simulink model "hdv_ctrl"  (R2026a)
settings: Solver=ode23tb  StopTime=simulation_length  MaxStep=tsample
undefined symbols (not defined in the file): available_torque, eta_v_m, eta_v_p, omega_e_rpm_ref, omega_l_max_rpm, R_tg, rpm, tau_load, tau_load_max, tsample, v_track1_ref, v_track2_ref
libraries: nesl_utility x20, fl_lib x13, linear_swashplate_ctrl_lib x4, variable_displacement_motor_lib x2, variable_displacement_pump_lib x2, flexshaft_lib x2, gear_lib x2, sl_discontinuities x2, engine_speed_ctrl_lib x1, engine_lib x1
settings Model: SimulationMode=accelerator  Creator=dbagn  LastModifiedBy=dbagn
settings SimscapeCC: SimscapeNominalValues="[{\"value\":\"1\",\"unit\":\"A\"},{\"value\":\"1\",\"unit\":\"bar\"},{\"value\":\"1\",\"unit\":\"cm^2\"},{\"value\":\"1\",\"unit\":\"cm^3/s\"},{\"value\":\"1\",\"unit\":\"kJ/kg\"},{\"value\":\"1\",\"unit\":\"kW\"},{\"value\":\"1\",\"unit\":\"l\"},{\"value\":\"1\",\"unit\":\"N\"},{\"value\":\"1\",\"unit\":\"N*m\"},{\"value\":\"1\",\"unit\":\"V\"}]"  SimscapeLogType=none  SimscapeLogDataHistory=5000.0

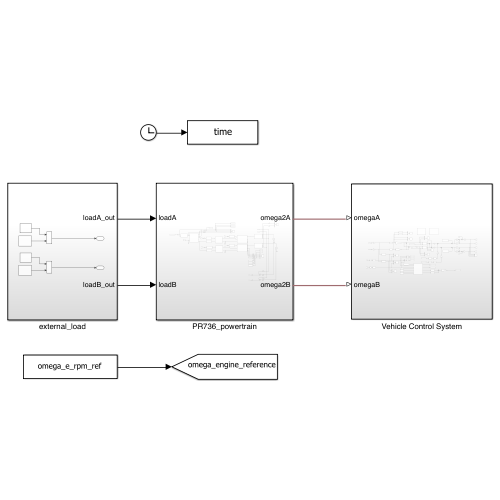
[thumbnail: Simulink's stored preview of the top-level diagram]
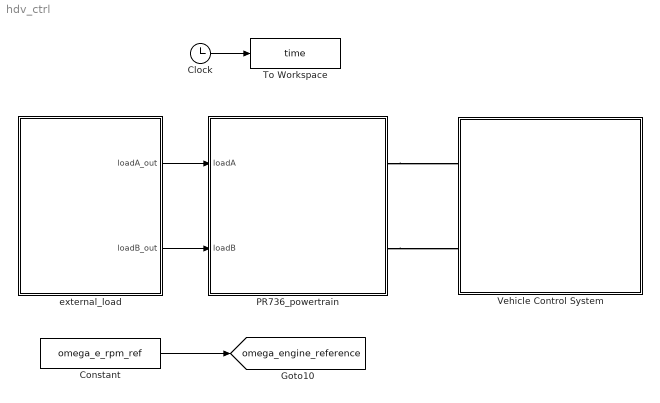
== system hdv_ctrl ==
  Clock : Clock
  Constant : Constant  Value=omega_e_rpm_ref
  PR736_powertrain : Subsystem
  To Workspace : ToWorkspace  VariableName=time  SampleTime=tsample
      settings: MaxDataPoints=Nsample
  Vehicle Control System : Subsystem
  external_load : Subsystem
  tag scope: omega_engine_reference=global
  wires:
  Clock/1 -> To Workspace/1
  Constant/1 -> [omega_engine_reference]
  external_load/2(loadB_out) -> PR736_powertrain/2(loadB)
  external_load/1(loadA_out) -> PR736_powertrain/1(loadA)
  connections:
  PR736_powertrain/RConn1 -- Vehicle Control System/LConn1
  PR736_powertrain/RConn2 -- Vehicle Control System/LConn2

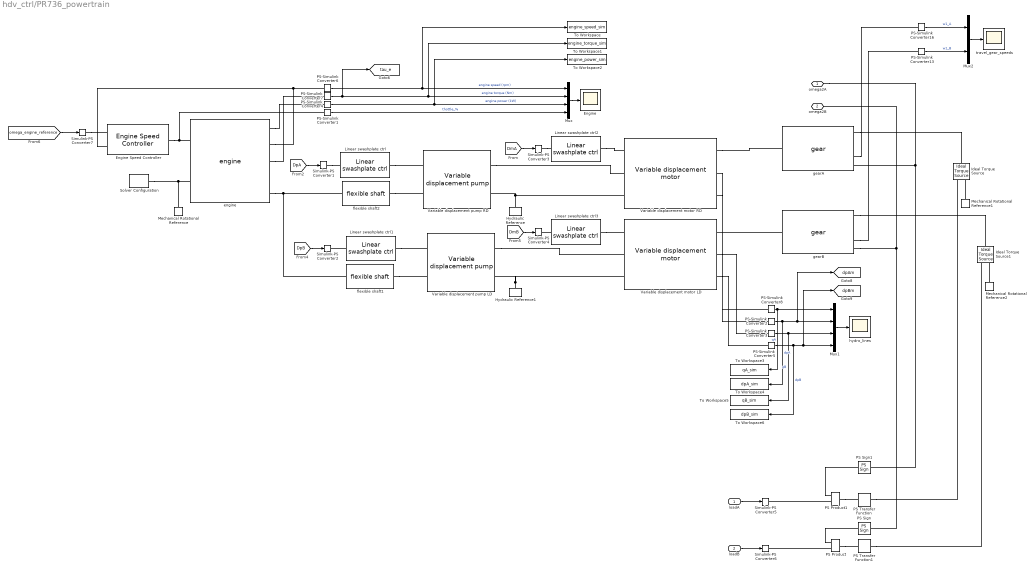
== system hdv_ctrl/PR736_powertrain ==
  loadA : Inport
  loadB : Inport  Port=2
  Engine : Scope
      settings: SampleTime=tsample  ActiveDisplayYMinimum=-336.80549  ActiveDisplayYMaximum=2213.60139
  Engine Speed Controller : engine_speed_ctrl_lib/Engine Speed Controller  kp=0.25 s  kint=2  kd=0 s^2  t_out_specify=off  t_out_priority=None  t_out=0  t_out_nominal_specify=off  t_out_nominal_unit=1  t_out_nominal_value=1
  Hydraulic Reference : fl_lib/Hydraulic/Hydraulic Elements/Hydraulic Reference
  Hydraulic Reference1 : fl_lib/Hydraulic/Hydraulic Elements/Hydraulic Reference
  Ideal Torque Source : fl_lib/Mechanical/Mechanical Sources/Ideal Torque Source
  Ideal Torque Source1 : fl_lib/Mechanical/Mechanical Sources/Ideal Torque Source
  Linear swashplate ctrl : linear_swashplate_ctrl_lib/Linear swashplate ctrl  a12=1 1/s  b2=1 1/m/s  k1=100 m  k2=20.5 m  N=10 m  kv=10  xv_specify=off  xv_priority=None  xv=0 m  xv_nominal_specify=off  xv_nominal_unit=m  xv_nominal_value=1  D1_specify=off  D1_priority=None  D1=0  D1_nominal_specify=off  D1_nominal_unit=1  D1_nominal_value=1  D2_specify=off  D2_priority=None  D2=0  D2_nominal_specify=off  D2_nominal_unit=1  D2_nominal_value=1
  Linear swashplate ctrl1 : linear_swashplate_ctrl_lib/Linear swashplate ctrl  a12=1 1/s  b2=1 1/m/s  k1=100 m  k2=20.5 m  N=10 m  kv=10  xv_specify=off  xv_priority=None  xv=0 m  xv_nominal_specify=off  xv_nominal_unit=m  xv_nominal_value=1  D1_specify=off  D1_priority=None  D1=0  D1_nominal_specify=off  D1_nominal_unit=1  D1_nominal_value=1  D2_specify=off  D2_priority=None  D2=0  D2_nominal_specify=off  D2_nominal_unit=1  D2_nominal_value=1
  Linear swashplate ctrl2 : linear_swashplate_ctrl_lib/Linear swashplate ctrl  a12=1 1/s  b2=1 1/m/s  k1=100 m  k2=20.5 m  N=5 m  kv=20  xv_specify=off  xv_priority=None  xv=0 m  xv_nominal_specify=off  xv_nominal_unit=m  xv_nominal_value=1  D1_specify=off  D1_priority=None  D1=0  D1_nominal_specify=off  D1_nominal_unit=1  D1_nominal_value=1  D2_specify=off  D2_priority=None  D2=0  D2_nominal_specify=off  D2_nominal_unit=1  D2_nominal_value=1
  Linear swashplate ctrl3 : linear_swashplate_ctrl_lib/Linear swashplate ctrl  a12=1 1/s  b2=1 1/m/s  k1=100 m  k2=20.5 m  N=5 m  kv=20  xv_specify=off  xv_priority=None  xv=0 m  xv_nominal_specify=off  xv_nominal_unit=m  xv_nominal_value=1  D1_specify=off  D1_priority=None  D1=0  D1_nominal_specify=off  D1_nominal_unit=1  D1_nominal_value=1  D2_specify=off  D2_priority=None  D2=0  D2_nominal_specify=off  D2_nominal_unit=1  D2_nominal_value=1
  Mechanical Rotational Reference : fl_lib/Mechanical/Rotational Elements/Mechanical Rotational Reference
  Mechanical Rotational Reference1 : fl_lib/Mechanical/Rotational Elements/Mechanical Rotational Reference
  Mechanical Rotational Reference2 : fl_lib/Mechanical/Rotational Elements/Mechanical Rotational Reference
  Mux : Mux
  Mux1 : Mux
  Mux2 : Mux  Inputs=2
  PS Product : fl_lib/Physical Signals/Functions/PS Product
  PS Product1 : fl_lib/Physical Signals/Functions/PS Product
  PS Sign : fl_lib/Physical Signals/Nonlinear Operators/PS Sign
  PS Sign1 : fl_lib/Physical Signals/Nonlinear Operators/PS Sign
  PS Transfer Function : fl_lib/Physical Signals/Linear Operators/PS Transfer Function  transfer_function_type=foundation.enum.transfer_function_type.lag  T=1 s  T1=2 s  T2=1 s  reset_method=foundation.enum.IntegratorResetSpec.None  initial_condition_spec=foundation.enum.IntegratorICSpec.Internal  y0=0 N*m
  PS Transfer Function1 : fl_lib/Physical Signals/Linear Operators/PS Transfer Function  transfer_function_type=foundation.enum.transfer_function_type.lag  T=1 s  T1=2 s  T2=1 s  reset_method=foundation.enum.IntegratorResetSpec.None  initial_condition_spec=foundation.enum.IntegratorICSpec.Internal  y0=0 N*m
  PS-Simulink Converter1 : nesl_utility/PS-Simulink Converter  PhysicalDomain=network_engine_domain  SubClassName=ps_output  LeftPortType=input  RightPortType=output  PseudoPeriodic=off  Frequencies=[]  VectorFormat=1-D array  Unit=inherit  AffineConversion=off
  PS-Simulink Converter13 : nesl_utility/PS-Simulink Converter  PhysicalDomain=network_engine_domain  SubClassName=ps_output  LeftPortType=input  RightPortType=output  PseudoPeriodic=off  Frequencies=[]  VectorFormat=1-D array  Unit=rpm  AffineConversion=on
  PS-Simulink Converter16 : nesl_utility/PS-Simulink Converter  PhysicalDomain=network_engine_domain  SubClassName=ps_output  LeftPortType=input  RightPortType=output  PseudoPeriodic=off  Frequencies=[]  VectorFormat=1-D array  Unit=rpm  AffineConversion=on
  PS-Simulink Converter2 : nesl_utility/PS-Simulink Converter  PhysicalDomain=network_engine_domain  SubClassName=ps_output  LeftPortType=input  RightPortType=output  PseudoPeriodic=off  Frequencies=[]  VectorFormat=1-D array  Unit=bar  AffineConversion=off
  PS-Simulink Converter3 : nesl_utility/PS-Simulink Converter  PhysicalDomain=network_engine_domain  SubClassName=ps_output  LeftPortType=input  RightPortType=output  PseudoPeriodic=off  Frequencies=[]  VectorFormat=1-D array  Unit=l/min  AffineConversion=off
  PS-Simulink Converter4 : nesl_utility/PS-Simulink Converter  PhysicalDomain=network_engine_domain  SubClassName=ps_output  LeftPortType=input  RightPortType=output  PseudoPeriodic=off  Frequencies=[]  VectorFormat=1-D array  Unit=kW  AffineConversion=off
  PS-Simulink Converter5 : nesl_utility/PS-Simulink Converter  PhysicalDomain=network_engine_domain  SubClassName=ps_output  LeftPortType=input  RightPortType=output  PseudoPeriodic=off  Frequencies=[]  VectorFormat=1-D array  Unit=bar  AffineConversion=off
  PS-Simulink Converter6 : nesl_utility/PS-Simulink Converter  PhysicalDomain=network_engine_domain  SubClassName=ps_output  LeftPortType=input  RightPortType=output  PseudoPeriodic=off  Frequencies=[]  VectorFormat=1-D array  Unit=rpm  AffineConversion=off
  PS-Simulink Converter7 : nesl_utility/PS-Simulink Converter  PhysicalDomain=network_engine_domain  SubClassName=ps_output  LeftPortType=input  RightPortType=output  PseudoPeriodic=off  Frequencies=[]  VectorFormat=1-D array  Unit=inherit  AffineConversion=off
  PS-Simulink Converter8 : nesl_utility/PS-Simulink Converter  PhysicalDomain=network_engine_domain  SubClassName=ps_output  LeftPortType=input  RightPortType=output  PseudoPeriodic=off  Frequencies=[]  VectorFormat=1-D array  Unit=l/min  AffineConversion=off
  Simulink-PS Converter{1..4} (4 alike) : nesl_utility/Simulink-PS Converter  PhysicalDomain=network_engine_domain  SubClassName=ps_input  LeftPortType=input  RightPortType=output  PseudoPeriodic=off  Frequencies=[]  NoiseDistribution=none  NoiseParameters=[]  Unit=1  AffineConversion=off  FilteringAndDerivatives=provide  SimscapeFilterOrder=1  InputFilterTimeConstant=0.001  UdotUserProvided=0
  Simulink-PS Converter5 : nesl_utility/Simulink-PS Converter  PhysicalDomain=network_engine_domain  SubClassName=ps_input  LeftPortType=input  RightPortType=output  PseudoPeriodic=off  Frequencies=[]  NoiseDistribution=none  NoiseParameters=[]  Unit=N*m  AffineConversion=off  FilteringAndDerivatives=provide  SimscapeFilterOrder=1  InputFilterTimeConstant=0.001  UdotUserProvided=0
  Simulink-PS Converter6 : nesl_utility/Simulink-PS Converter  PhysicalDomain=network_engine_domain  SubClassName=ps_input  LeftPortType=input  RightPortType=output  PseudoPeriodic=off  Frequencies=[]  NoiseDistribution=none  NoiseParameters=[]  Unit=N*m  AffineConversion=off  FilteringAndDerivatives=provide  SimscapeFilterOrder=1  InputFilterTimeConstant=0.001  UdotUserProvided=0
  Simulink-PS Converter7 : nesl_utility/Simulink-PS Converter  PhysicalDomain=network_engine_domain  SubClassName=ps_input  LeftPortType=input  RightPortType=output  PseudoPeriodic=off  Frequencies=[]  NoiseDistribution=none  NoiseParameters=[]  Unit=rpm  AffineConversion=off  FilteringAndDerivatives=provide  SimscapeFilterOrder=1  InputFilterTimeConstant=0.001  UdotUserProvided=0
  Solver Configuration : nesl_utility/Solver Configuration  PhysicalDomain=network_engine_domain  SubClassName=solver  LeftPortType=input  RightPortType=generic  Tones=[]  Harmonics=[]  SimulateNoise=off  Profile=off  UseLocalSampling=off  EnableSwitchedLinearOptims=on  FrequencyDomain=off  UseCCode=off  RelTol=0.001  AbsTol=1e-06  MinStep=1e-09  ToWorkspace=off  RevertToSquareIcSolve=off  NumHomotopyIterations=100  PhasorMode=off  PhasorModeNumHarmonics=1  ConsistencySolver=NEWTON_FTOL  CanonicalOrdering=UNORDERED  OptimizeIntermediates=UNOPTIMIZED  IndexReductionMethod=DerivativeReplacement  DoDC=off  ResidualTolerance=1e-09  ConsistencyTolSource=GLOBAL  ConsistencyAbsTol=0.001  ConsistencyRelTol=0.001  ConsistencyTolFactor=0.001  UseLocalSolver=on  LocalSolverChoice=NE_BACKWARD_EULER_ADVANCER  ResolveIndetEquations=on  FunctionEvalNumThread=1  LocalSolverSampleTime=tsample  DoFixedCost=on  MaxNonlinIter=3  MaxModeIter=2  ComputeImpulses=off  ImpulseIterations=2  LinearAlgebra=auto  LinearAlgebraNumThread=0  EquationFormulation=NE_TIME_EF  DelaysMemoryBudget=1024  AutomaticFiltering=on  FilteringTimeConstant=tsample  PartitionStorageMethod=AS_NEEDED  PartitionMemoryBudget=1024  PartitionMethod=ROBUST  MultibodyUseLocalSolver=off  MultibodyLocalSolverChoice=ODE1  MultibodyLocalSolverSampleTime=0.001
  To Workspace : ToWorkspace  VariableName=engine_speed_sim  SampleTime=tsample
      settings: MaxDataPoints=Nsample
  To Workspace1 : ToWorkspace  VariableName=engine_torque_sim  SampleTime=tsample
      settings: MaxDataPoints=Nsample
  To Workspace2 : ToWorkspace  VariableName=engine_power_sim  SampleTime=tsample
      settings: MaxDataPoints=Nsample
  To Workspace3 : ToWorkspace  VariableName=qA_sim  SampleTime=tsample
      settings: MaxDataPoints=Nsample
  To Workspace4 : ToWorkspace  VariableName=dpA_sim  SampleTime=tsample
      settings: MaxDataPoints=Nsample
  To Workspace5 : ToWorkspace  VariableName=qB_sim  SampleTime=tsample
      settings: MaxDataPoints=Nsample
  To Workspace6 : ToWorkspace  VariableName=dpB_sim  SampleTime=tsample
      settings: MaxDataPoints=Nsample
  Variable displacement motor LD : variable_displacement_motor_lib/Variable displacement motor  max_Dv=Vm_nom cm^3/rev  min_Dv=20 cm^3/rev  inertia_motor=0.0402 kg*m^2  oil_vol=4.1 l  bp=1 N*m/(rad/s)  lk=1e-6 m  t_specify=off  t_priority=None  t=0 N*m  t_nominal_specify=off  t_nominal_value=1  t_nominal_unit=N*m  q_specify=off  q_priority=None  q=0 m^3/s  q_nominal_specify=off  q_nominal_value=1  q_nominal_unit=m^3/s  qt_specify=off  qt_priority=None  qt=0 m^3/s  qt_nominal_specify=off  qt_nominal_value=1  qt_nominal_unit=m^3/s  qleak_specify=off  qleak_priority=None  qleak=0 m^3/s  qleak_nominal_specify=off  qleak_nominal_value=1  qleak_nominal_unit=m^3/s  Dv_specify=off  Dv_priority=None  Dv=0 cm^3/rev  Dv_nominal_specify=off  Dv_nominal_value=1  Dv_nominal_unit=cm^3/rev  dp_specify=off  dp_priority=None  dp=0 Pa  dp_nominal_specify=off  dp_nominal_value=1  dp_nominal_unit=Pa  wm_specify=off  wm_priority=None  wm=0 rad/s  wm_nominal_specify=off  wm_nominal_value=1  wm_nominal_unit=rad/s
  Variable displacement motor RD : variable_displacement_motor_lib/Variable displacement motor  max_Dv=Vm_nom cm^3/rev  min_Dv=20 cm^3/rev  inertia_motor=0.0402 kg*m^2  oil_vol=4.1 l  bp=1 N*m/(rad/s)  lk=1e-6 m  t_specify=off  t_priority=None  t=0 N*m  t_nominal_specify=off  t_nominal_value=1  t_nominal_unit=N*m  q_specify=off  q_priority=None  q=0 m^3/s  q_nominal_specify=off  q_nominal_value=1  q_nominal_unit=m^3/s  qt_specify=off  qt_priority=None  qt=0 m^3/s  qt_nominal_specify=off  qt_nominal_value=1  qt_nominal_unit=m^3/s  qleak_specify=off  qleak_priority=None  qleak=0 m^3/s  qleak_nominal_specify=off  qleak_nominal_value=1  qleak_nominal_unit=m^3/s  Dv_specify=off  Dv_priority=None  Dv=0 cm^3/rev  Dv_nominal_specify=off  Dv_nominal_value=1  Dv_nominal_unit=cm^3/rev  dp_specify=off  dp_priority=None  dp=0 Pa  dp_nominal_specify=off  dp_nominal_value=1  dp_nominal_unit=Pa  wm_specify=off  wm_priority=None  wm=0 rad/s  wm_nominal_specify=off  wm_nominal_value=1  wm_nominal_unit=rad/s
  Variable displacement pump LD : variable_displacement_pump_lib/Variable displacement pump  max_Dv=Vp_nom cm^3/rev  inertia_pump=0.027 kg*m^2  oil_vol=3.0 l  bp=1 N*m/(rad/s)  lk=1e-6 m  t_specify=off  t_priority=None  t=0 N*m  t_nominal_specify=off  t_nominal_value=1  t_nominal_unit=N*m  q_specify=off  q_priority=None  q=0 m^3/s  q_nominal_specify=off  q_nominal_value=1  q_nominal_unit=m^3/s  qt_specify=off  qt_priority=None  qt=0 m^3/s  qt_nominal_specify=off  qt_nominal_value=1  qt_nominal_unit=m^3/s  qleak_specify=off  qleak_priority=None  qleak=0 m^3/s  qleak_nominal_specify=off  qleak_nominal_value=1  qleak_nominal_unit=m^3/s  Dv_specify=off  Dv_priority=None  Dv=0 cm^3/rev  Dv_nominal_specify=off  Dv_nominal_value=1  Dv_nominal_unit=cm^3/rev  dp_specify=off  dp_priority=None  dp=0 Pa  dp_nominal_specify=off  dp_nominal_value=1  dp_nominal_unit=Pa  we_specify=off  we_priority=None  we=0 rad/s  we_nominal_specify=off  we_nominal_value=1  we_nominal_unit=rad/s
  Variable displacement pump RD : variable_displacement_pump_lib/Variable displacement pump  max_Dv=Vp_nom cm^3/rev  inertia_pump=0.027 kg*m^2  oil_vol=3.0 l  bp=1 N*m/(rad/s)  lk=1e-6 m  t_specify=off  t_priority=None  t=0 N*m  t_nominal_specify=off  t_nominal_value=1  t_nominal_unit=N*m  q_specify=off  q_priority=None  q=0 m^3/s  q_nominal_specify=off  q_nominal_value=1  q_nominal_unit=m^3/s  qt_specify=off  qt_priority=None  qt=0 m^3/s  qt_nominal_specify=off  qt_nominal_value=1  qt_nominal_unit=m^3/s  qleak_specify=off  qleak_priority=None  qleak=0 m^3/s  qleak_nominal_specify=off  qleak_nominal_value=1  qleak_nominal_unit=m^3/s  Dv_specify=off  Dv_priority=None  Dv=0 cm^3/rev  Dv_nominal_specify=off  Dv_nominal_value=1  Dv_nominal_unit=cm^3/rev  dp_specify=off  dp_priority=None  dp=0 Pa  dp_nominal_specify=off  dp_nominal_value=1  dp_nominal_unit=Pa  we_specify=off  we_priority=None  we=0 rad/s  we_nominal_specify=off  we_nominal_value=1  we_nominal_unit=rad/s
  engine : engine_lib/engine  dynamic_response=simscape.enum.onoff.off  cshaft_inertia=5.00 kg*m^2  initial_speed=1
  flexible shaft1 : flexshaft_lib/flexible shaft  b1=b1 N*m/(rad/s)  J1=J1 kg*m^2  b2=b2 N*m/(rad/s)  J2=J2 kg*m^2  b_theta=b_theta N*m/(rad/s)  k_theta=k_theta N*m/rad  w_1_specify=off  w_1_priority=None  w_1=0 rad/s  w_1_nominal_specify=off  w_1_nominal_value=1  w_1_nominal_unit=rad/s  w_2_specify=off  w_2_priority=None  w_2=0 rad/s  w_2_nominal_specify=off  w_2_nominal_value=1  w_2_nominal_unit=rad/s  t_1_specify=off  t_1_priority=None  t_1=0 N*m  t_1_nominal_specify=off  t_1_nominal_value=1  t_1_nominal_unit=N*m  t_2_specify=off  t_2_priority=None  t_2=0 N*m  t_2_nominal_specify=off  t_2_nominal_value=1  t_2_nominal_unit=N*m  t_theta_specify=off  t_theta_priority=None  t_theta=0 N*m  t_theta_nominal_specify=off  t_theta_nominal_value=1  t_theta_nominal_unit=N*m
  flexible shaft2 : flexshaft_lib/flexible shaft  b1=b1 N*m/(rad/s)  J1=J1 kg*m^2  b2=b2 N*m/(rad/s)  J2=J2 kg*m^2  b_theta=b_theta N*m/(rad/s)  k_theta=k_theta N*m/rad  w_1_specify=off  w_1_priority=None  w_1=0 rad/s  w_1_nominal_specify=off  w_1_nominal_value=1  w_1_nominal_unit=rad/s  w_2_specify=off  w_2_priority=None  w_2=0 rad/s  w_2_nominal_specify=off  w_2_nominal_value=1  w_2_nominal_unit=rad/s  t_1_specify=off  t_1_priority=None  t_1=0 N*m  t_1_nominal_specify=off  t_1_nominal_value=1  t_1_nominal_unit=N*m  t_2_specify=off  t_2_priority=None  t_2=0 N*m  t_2_nominal_specify=off  t_2_nominal_value=1  t_2_nominal_unit=N*m  t_theta_specify=off  t_theta_priority=None  t_theta=0 N*m  t_theta_nominal_specify=off  t_theta_nominal_value=1  t_theta_nominal_unit=N*m
  gearA : gear_lib/gear  n1=n_tg  n2=1  b1=0.02 N*m/(rad/s)  J1=0.25 kg*m^2  b2=track_friction_1 N*m/(rad/s)  J2=2 kg*m^2  k_theta_1=k_theta N*m/rad  w_1_specify=off  w_1_priority=None  w_1=0 rad/s  w_1_nominal_specify=off  w_1_nominal_unit=rad/s  w_1_nominal_value=1  w_2_specify=off  w_2_priority=None  w_2=0 rad/s  w_2_nominal_specify=off  w_2_nominal_unit=rad/s  w_2_nominal_value=1  t_1_specify=off  t_1_priority=None  t_1=0 N*m  t_1_nominal_specify=off  t_1_nominal_unit=N*m  t_1_nominal_value=1  t_2_specify=off  t_2_priority=None  t_2=0 N*m  t_2_nominal_specify=off  t_2_nominal_unit=N*m  t_2_nominal_value=1  t_theta_1_specify=off  t_theta_1_priority=None  t_theta_1=0 N*m  t_theta_1_nominal_specify=off  t_theta_1_nominal_unit=N*m  t_theta_1_nominal_value=1  t_theta_2_specify=off  t_theta_2_priority=None  t_theta_2=0 N*m  t_theta_2_nominal_specify=off  t_theta_2_nominal_unit=N*m  t_theta_2_nominal_value=1
  gearB : gear_lib/gear  n1=n_tg  n2=1  b1=0.02 N*m/(rad/s)  J1=0.25 kg*m^2  b2=track_friction_2 N*m/(rad/s)  J2=2 kg*m^2  k_theta_1=k_theta N*m/rad  w_1_specify=off  w_1_priority=None  w_1=0 rad/s  w_1_nominal_specify=off  w_1_nominal_unit=rad/s  w_1_nominal_value=1  w_2_specify=off  w_2_priority=None  w_2=0 rad/s  w_2_nominal_specify=off  w_2_nominal_unit=rad/s  w_2_nominal_value=1  t_1_specify=off  t_1_priority=None  t_1=0 N*m  t_1_nominal_specify=off  t_1_nominal_unit=N*m  t_1_nominal_value=1  t_2_specify=off  t_2_priority=None  t_2=0 N*m  t_2_nominal_specify=off  t_2_nominal_unit=N*m  t_2_nominal_value=1  t_theta_1_specify=off  t_theta_1_priority=None  t_theta_1=0 N*m  t_theta_1_nominal_specify=off  t_theta_1_nominal_unit=N*m  t_theta_1_nominal_value=1  t_theta_2_specify=off  t_theta_2_priority=None  t_theta_2=0 N*m  t_theta_2_nominal_specify=off  t_theta_2_nominal_unit=N*m  t_theta_2_nominal_value=1
  hydro_lines : Scope
      settings: SampleTime=tsample  ActiveDisplayYMinimum=-45.39714  ActiveDisplayYMaximum=408.5743
  travel_gear_speeds : Scope
      settings: SampleTime=tsample  ActiveDisplayYMinimum=-2096.53273  ActiveDisplayYMaximum=232.94808  DataLoggingVariableName=ScopeData3
  omega2A : PMIOPort  Side=Right
  omega2B : PMIOPort  Port=2  Side=Right
  tag scope: dpAm=global, dpBm=global, tau_e=global
  wires:
  PS-Simulink Converter7/1 -> [tau_e], To Workspace1/1, Mux/2  "engine torque (Nm)"
  Mux1/1 -> hydro_lines/1
  PS-Simulink Converter5/1 -> To Workspace6/1, Mux1/4, [dpBm]  "dpB"
  PS-Simulink Converter8/1 -> To Workspace3/1, Mux1/1  "qA"
  [DmB] -> Simulink-PS Converter4/1
  PS-Simulink Converter6/1 -> To Workspace/1, Mux/1  "engine speed (rpm)"
  PS-Simulink Converter3/1 -> To Workspace5/1, Mux1/3  "qB"
  Mux/1 -> Engine/1
  [DpA] -> Simulink-PS Converter1/1
  PS-Simulink Converter2/1 -> To Workspace4/1, Mux1/2, [dpAm]  "dpA"
  [DmA] -> Simulink-PS Converter3/1
  [DpB] -> Simulink-PS Converter2/1
  PS-Simulink Converter1/1 -> Mux/4  "thottle_%"
  PS-Simulink Converter4/1 -> Mux/3, To Workspace2/1  "engine power (kW)"
  [omega_engine_reference] -> Simulink-PS Converter7/1
  loadA/1 -> Simulink-PS Converter5/1
  loadB/1 -> Simulink-PS Converter6/1
  PS-Simulink Converter13/1 -> Mux2/2  "w1_B"
  PS-Simulink Converter16/1 -> Mux2/1  "w1_A"
  Mux2/1 -> travel_gear_speeds/1
  connections:
  Engine Speed Controller/RConn1 -- engine/LConn1 -- PS-Simulink Converter1/LConn1
  engine/RConn1 -- PS-Simulink Converter4/LConn1
  Linear swashplate ctrl1/LConn1 -- Simulink-PS Converter2/RConn1
  Linear swashplate ctrl1/RConn1 -- Variable displacement pump LD/LConn1
  Variable displacement pump RD/RConn1 -- Variable displacement motor RD/LConn2
  Simulink-PS Converter7/RConn1 -- Engine Speed Controller/LConn1
  engine/RConn2 -- Engine Speed Controller/LConn2 -- PS-Simulink Converter6/LConn1
  Variable displacement pump LD/RConn1 -- Variable displacement motor LD/LConn2
  flexible shaft1/RConn1 -- Variable displacement pump LD/LConn2
  Mechanical Rotational Reference/LConn1 -- Solver Configuration/RConn1 -- engine/LConn2
  Mechanical Rotational Reference1/LConn1 -- Ideal Torque Source/RConn2
  flexible shaft2/RConn1 -- Variable displacement pump RD/LConn2
  Hydraulic Reference1/LConn1 -- Variable displacement pump LD/RConn2 -- Variable displacement motor LD/LConn3
  flexible shaft2/LConn1 -- flexible shaft1/LConn1 -- engine/RConn5
  PS Sign1/RConn1 -- PS Product1/LConn1
  Linear swashplate ctrl3/RConn1 -- Variable displacement motor LD/LConn1
  Linear swashplate ctrl/RConn1 -- Variable displacement pump RD/LConn1
  gearB/LConn1 -- Variable displacement motor LD/RConn1
  Variable displacement motor LD/RConn2 -- PS-Simulink Converter3/LConn1
  Linear swashplate ctrl2/RConn1 -- Variable displacement motor RD/LConn1
  Variable displacement motor RD/LConn3 -- Hydraulic Reference/LConn1 -- Variable displacement pump RD/RConn2
  Linear swashplate ctrl3/LConn1 -- Simulink-PS Converter4/RConn1
  Simulink-PS Converter1/RConn1 -- Linear swashplate ctrl/LConn1
  gearB/RConn5 -- omega2B/RConn1 -- PS Sign/LConn1
  Variable displacement motor RD/RConn3 -- PS-Simulink Converter2/LConn1
  engine/RConn3 -- PS-Simulink Converter7/LConn1
  Mechanical Rotational Reference2/LConn1 -- Ideal Torque Source1/RConn2
  PS Product/LConn2 -- Simulink-PS Converter6/RConn1
  PS Transfer Function/RConn1 -- Ideal Torque Source/RConn1
  omega2A/RConn1 -- gearA/RConn5 -- PS Sign1/LConn1
  PS Product/RConn1 -- PS Transfer Function1/LConn1
  PS Sign/RConn1 -- PS Product/LConn1
  Simulink-PS Converter3/RConn1 -- Linear swashplate ctrl2/LConn1
  Variable displacement motor RD/RConn1 -- gearA/LConn1
  Variable displacement motor LD/RConn3 -- PS-Simulink Converter5/LConn1
  Variable displacement motor RD/RConn2 -- PS-Simulink Converter8/LConn1
  PS Product1/RConn1 -- PS Transfer Function/LConn1
  PS Transfer Function1/RConn1 -- Ideal Torque Source1/RConn1
  PS Product1/LConn2 -- Simulink-PS Converter5/RConn1
  gearB/RConn4 -- PS-Simulink Converter13/LConn1
  gearA/RConn4 -- PS-Simulink Converter16/LConn1
  gearA/RConn1 -- Ideal Torque Source/LConn1
  gearB/RConn1 -- Ideal Torque Source1/LConn1

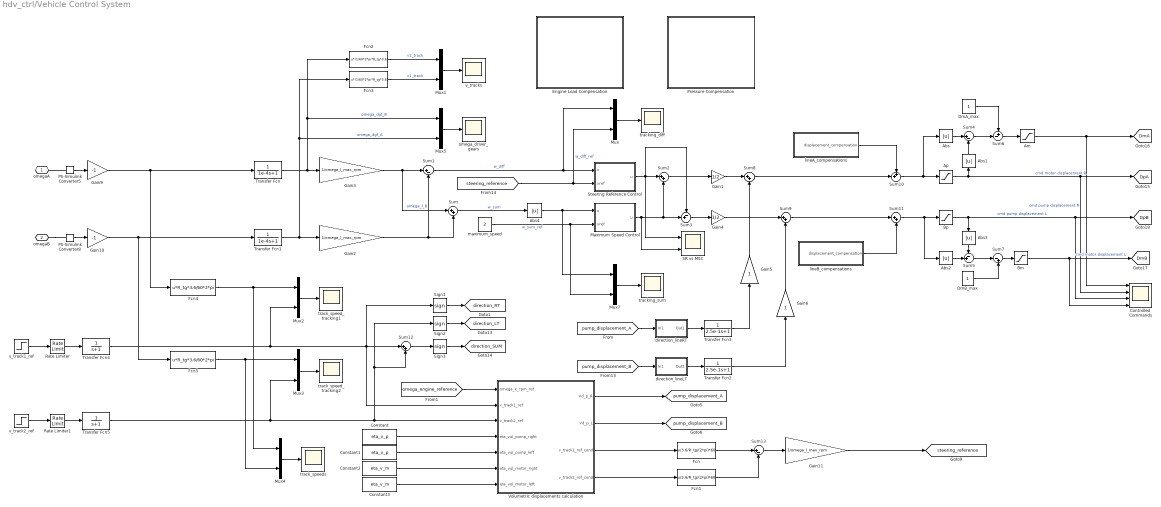
== system hdv_ctrl/Vehicle Control System ==
  Abs{,1..4} (5 alike) : Abs  SaturateOnIntegerOverflow=off
  Am : Saturate  UpperLimit=1  LowerLimit=0.36
  Ap : Saturate  UpperLimit=1  LowerLimit=-1
  Bm : Saturate  UpperLimit=1  LowerLimit=0.36
  Bp : Saturate  UpperLimit=1  LowerLimit=-1
  Constant : Constant  Value=eta_v_p
  Constant1 : Constant  Value=eta_v_p
  Constant2 : Constant  Value=eta_v_m
  Constant3 : Constant  Value=eta_v_m
  Controlled Commands : Scope  NumInputPorts=4
      settings: SampleTime=tsample  ActiveDisplayYMinimum=-0.1826  ActiveDisplayYMaximum=1.1314  DataLoggingVariableName=ScopeData5
  DmA_max : Constant
  DmB_max : Constant
  Engine Load Compensation : Subsystem
  Fcn : Fcn  Expr=u/3.6/R_tg/(2*pi)*60
  Fcn1 : Fcn  Expr=u/3.6/R_tg/(2*pi)*60
  Fcn2 : Fcn  Expr=u*(1/60*2*pi*R_tg*3.6)
  Fcn3 : Fcn  Expr=u*(1/60*2*pi*R_tg*3.6)
  Fcn4 : Fcn  Expr=u*R_tg*3.6/60*2*pi
  Fcn5 : Fcn  Expr=u*R_tg*3.6/60*2*pi
  Gain1 : Gain  Gain=1/2
  Gain10 : Gain  Gain=-1
  Gain11 : Gain  Gain=1/omega_l_max_rpm
  Gain2 : Gain  Gain=1/omega_l_max_rpm
  Gain3 : Gain  Gain=1/omega_l_max_rpm
  Gain4 : Gain  Gain=1/2
  Gain5 : Gain
  Gain6 : Gain
  Gain9 : Gain  Gain=-1
  Maximum Speed Control : Subsystem  mask{kp=0.25, ki=4, ts=tsample, sat_pos=0, sat_neg=-3.28}
  Mux{,1..5,7} (7 alike) : Mux  Inputs=2
  PS-Simulink Converter5 : nesl_utility/PS-Simulink Converter  PhysicalDomain=network_engine_domain  SubClassName=ps_output  LeftPortType=input  RightPortType=output  PseudoPeriodic=off  Frequencies=[]  VectorFormat=1-D array  Unit=rpm  AffineConversion=off
  PS-Simulink Converter8 : nesl_utility/PS-Simulink Converter  PhysicalDomain=network_engine_domain  SubClassName=ps_output  LeftPortType=input  RightPortType=output  PseudoPeriodic=off  Frequencies=[]  VectorFormat=1-D array  Unit=rpm  AffineConversion=off
  Pressure Compensation : Subsystem
  Rate Limiter : RateLimiter  RisingSlewLimit=v_track1_ref/4  FallingSlewLimit=-v_track1_ref/4  SampleTimeMode=inherited
  Rate Limiter1 : RateLimiter  RisingSlewLimit=v_track2_ref/4  FallingSlewLimit=-v_track2_ref/4  SampleTimeMode=inherited
  SR vs MSC : Scope  NumInputPorts=2
      settings: SampleTime=tsample  ActiveDisplayYMinimum=-9E-16  ActiveDisplayYMaximum=7E-16  DataLoggingVariableName=ScopeData6
  Sign1 : Signum
  Sign2 : Signum
  Sign3 : Signum
  Steering Reference Control : Subsystem  mask{kp=0.5, ki=8, ts=tsample, sat_pos=3.28, sat_neg=-3.28}
  Sum{,2,8..9,11..12} (6 alike) : Sum  Inputs=|++
  Sum1 : Sum  Inputs=|+-
  Sum10 : Sum  Inputs=++|
  Sum13 : Sum  Inputs=|+-
  Sum3 : Sum  Inputs=-+|
  Sum4 : Sum  Inputs=|+-
  Sum5 : Sum  Inputs=-+|
  Sum6 : Sum  Inputs=+-|
  Sum7 : Sum  Inputs=|-+
  Transfer Fcn : TransferFcn  Denominator=[1e-4 1]
  Transfer Fcn1 : TransferFcn  Denominator=[1e-4 1]
  Transfer Fcn2 : TransferFcn  Denominator=[2.5e-1 1]
  Transfer Fcn3 : TransferFcn  Denominator=[2.5e-1 1]
  Transfer Fcn4 : TransferFcn  Denominator=[1 1]
  Transfer Fcn5 : TransferFcn  Denominator=[1 1]
  Volumetric displacements calculation : MATLAB Function  TreatAsAtomicUnit=on
  direction_lineLT : Subsystem
  direction_lineRT : Subsystem
  lineA_compensations : Subsystem
  "lineB_compensations " : Subsystem
  maximum_speed : Constant  Value=2
  omega_driver_gears : Scope
      settings: SampleTime=tsample  ActiveDisplayYMinimum=-6.02093  ActiveDisplayYMaximum=54.1884  DataLoggingVariableName=ScopeData5
  track_speed_tracking1 : Scope
      settings: SampleTime=tsample  ActiveDisplayYMinimum=-6.02093  ActiveDisplayYMaximum=54.1884
  track_speed_tracking2 : Scope
      settings: SampleTime=tsample  ActiveDisplayYMinimum=-6.02093  ActiveDisplayYMaximum=54.1884  DataLoggingVariableName=ScopeData2
  track_speeds : Scope
      settings: SampleTime=tsample  ActiveDisplayYMinimum=-6.02093  ActiveDisplayYMaximum=54.1884  DataLoggingVariableName=ScopeData3
  tracking_diff : Scope
      settings: SampleTime=tsample  ActiveDisplayYMinimum=-0.07331  ActiveDisplayYMaximum=0.0086  DataLoggingVariableName=ScopeData2
  tracking_sum : Scope
      settings: SampleTime=tsample  ActiveDisplayYMinimum=-0.33251  ActiveDisplayYMaximum=2.25917
  v_track1_ref : Step  Time=10  FinalValue=v_track1_ref  SampleTime=0
  v_track2_ref : Step  Time=10  FinalValue=v_track2_ref  SampleTime=0
  v_tracks : Scope
      settings: SampleTime=tsample  ActiveDisplayYMinimum=-1  ActiveDisplayYMaximum=9
  omegaA : PMIOPort  Side=Left
  omegaB : PMIOPort  Port=2  Side=Left
  tag scope: DmA=global, DmB=global, DpA=global, DpB=global, direction_LT=global, direction_RT=global, direction_SUM=global, pump_displacement_A=global, pump_displacement_B=global, steering_reference=global
  wires:
  Mux/1 -> tracking_diff/1
  [steering_reference] -> Mux/2, Steering Reference Control/2(xref)  "w_diff_ref"
  Sum2/1 -> Gain1/1
  Gain3/1 -> Sum/1, Sum1/1
  Gain2/1 -> Sum1/2, Sum/2  "omega_l_B"
  Sum3/1 -> Gain4/1
  Sum4/1 -> Sum6/2
  DmA_max/1 -> Sum6/1
  Sum6/1 -> Am/1
  DmB_max/1 -> Sum7/2
  Sum5/1 -> Sum7/1
  Sum7/1 -> Bm/1
  Mux5/1 -> omega_driver_gears/1
  Sum1/1 -> Mux/1, Steering Reference Control/1(x)  "w_diff"
  [pump_displacement_B] -> direction_lineLT/1(In1)
  Gain1/1 -> Sum8/1
  Gain4/1 -> Sum9/1
  Maximum Speed Control/1(u) -> SR vs MSC/2, Sum2/2, Sum3/2
  Sum/1 -> Abs4/1  "w_sum"
  Mux7/1 -> tracking_sum/1
  [pump_displacement_A] -> direction_lineRT/1(In1)
  Abs/1 -> Sum4/1
  Abs1/1 -> Sum4/2
  Abs2/1 -> Sum5/2
  Abs3/1 -> Sum5/1
  Sum8/1 -> Sum10/2
  Sum9/1 -> Sum11/1
  maximum_speed/1 -> Maximum Speed Control/2(xref), Mux7/2  "w_sum_ref"
  Sum10/1 -> Abs/1, Ap/1
  Sum11/1 -> Bp/1, Abs2/1
  Volumetric displacements calculation/1(Vd_p_R) -> [pump_displacement_A]
  Volumetric displacements calculation/2(Vd_p_L) -> [pump_displacement_B]
  lineA_compensations/1(displacement_compensation) -> Sum10/1
  "lineB_compensations "/1(displacement_compensation) -> Sum11/2
  Fcn/1 -> Sum13/1
  Fcn1/1 -> Sum13/2
  Sum13/1 -> Gain11/1
  Transfer Fcn4/1 -> Mux2/2, Volumetric displacements calculation/2(v_track1_ref), Sum12/1, Sign1/1
  Bp/1 -> [DpB], Controlled Commands/3, Abs3/1  "cmd pump displacement L"
  Ap/1 -> [DpA], Controlled Commands/2, Abs1/1  "cmd pump displacement R"
  Am/1 -> [DmA], Controlled Commands/1  "cmd motor displacement R"
  Bm/1 -> [DmB], Controlled Commands/4  "cmd motor displacement L"
  [omega_engine_reference] -> Volumetric displacements calculation/1(omega_e_rpm_ref)
  Constant3/1 -> Volumetric displacements calculation/7(eta_vol_motor_left)
  Constant2/1 -> Volumetric displacements calculation/6(eta_vol_motor_right)
  Constant1/1 -> Volumetric displacements calculation/5(eta_vol_pump_left)
  Constant/1 -> Volumetric displacements calculation/4(eta_vol_pump_right)
  Sign1/1 -> [direction_RT]
  Steering Reference Control/1(u) -> Sum3/1, SR vs MSC/1, Sum2/1
  Transfer Fcn3/1 -> Gain5/1
  Transfer Fcn2/1 -> Gain6/1
  Abs4/1 -> Mux7/1, Maximum Speed Control/1(x)
  Sign2/1 -> [direction_LT]
  Sum12/1 -> Sign3/1
  Sign3/1 -> [direction_SUM]
  Gain11/1 -> [steering_reference]
  Volumetric displacements calculation/3(v_track1_ref_cond) -> Fcn/1
  Volumetric displacements calculation/4(v_track2_ref_cond) -> Fcn1/1
  direction_lineRT/1(Out1) -> Transfer Fcn3/1
  direction_lineLT/1(Out1) -> Transfer Fcn2/1
  Gain5/1 -> Sum8/2
  Gain6/1 -> Sum9/2
  Gain10/1 -> Fcn5/1, Transfer Fcn1/1
  Gain9/1 -> Fcn4/1, Transfer Fcn/1
  PS-Simulink Converter8/1 -> Gain10/1
  PS-Simulink Converter5/1 -> Gain9/1
  Mux1/1 -> v_tracks/1
  Transfer Fcn/1 -> Fcn2/1, Mux5/1, Gain3/1  "omega_dgf_B"
  Transfer Fcn1/1 -> Fcn3/1, Mux5/2, Gain2/1  "omega_dgf_A"
  Fcn2/1 -> Mux1/1  "v2_track"
  Fcn3/1 -> Mux1/2  "v1_track"
  v_track1_ref/1 -> Rate Limiter/1
  Rate Limiter/1 -> Transfer Fcn4/1
  v_track2_ref/1 -> Rate Limiter1/1
  Rate Limiter1/1 -> Transfer Fcn5/1
  Mux2/1 -> track_speed_tracking1/1
  Fcn4/1 -> Mux4/1, Mux2/1
  Fcn5/1 -> Mux4/2, Mux3/1
  Mux3/1 -> track_speed_tracking2/1
  Transfer Fcn5/1 -> Mux3/2, Sign2/1, Sum12/2, Volumetric displacements calculation/3(v_track2_ref)
  Mux4/1 -> track_speeds/1
  connections:
  omegaB/RConn1 -- PS-Simulink Converter8/LConn1
  PS-Simulink Converter5/LConn1 -- omegaA/RConn1

== system hdv_ctrl/external_load ==
  Product1 : Product
  Product3 : Product
  Q1 : Constant  Value=-1
  Q2 : Constant  Value=-1
  loadA : Subsystem
  loadB : Subsystem
  loadA_out : Outport
  loadB_out : Outport  Port=2
  wires:
  loadB/1(Out1) -> Product3/2
  loadA/1(Out1) -> Product1/2
  Q2/1 -> Product3/1
  Q1/1 -> Product1/1
  Product1/1 -> loadA_out/1
  Product3/1 -> loadB_out/1

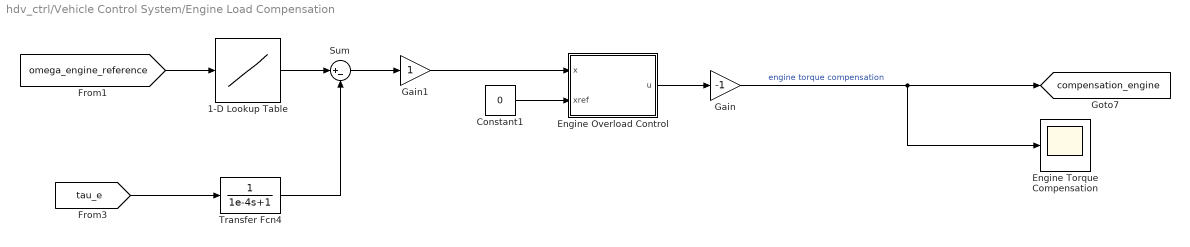
== system hdv_ctrl/Vehicle Control System/Engine Load Compensation ==
  1-D Lookup Table : Lookup_n-D  NumberOfTableDimensions=1  BreakpointsForDimension1=rpm  Table=available_torque  InternalRulePriority=Speed  RndMeth=Simplest
  Constant1 : Constant  Value=0
  Engine Overload Control : Subsystem  mask{kp=5/1500, ki=18/1500, ts=tsample, sat_pos=1.64, sat_neg=0}
  Engine Torque Compensation : Scope
      settings: SampleTime=tsample  ActiveDisplayYMinimum=-1.845  ActiveDisplayYMaximum=0.205  DataLoggingVariableName=ScopeData4
  Gain : Gain  Gain=-1
  Gain1 : Gain
  Sum : Sum  Inputs=|+-
  Transfer Fcn4 : TransferFcn  Denominator=[1e-4 1]
  tag scope: compensation_engine=global
  wires:
  Transfer Fcn4/1 -> Sum/2
  1-D Lookup Table/1 -> Sum/1
  Engine Overload Control/1(u) -> Gain/1
  [omega_engine_reference] -> 1-D Lookup Table/1
  [tau_e] -> Transfer Fcn4/1
  Sum/1 -> Gain1/1
  Constant1/1 -> Engine Overload Control/2(xref)
  Gain1/1 -> Engine Overload Control/1(x)
  Gain/1 -> Engine Torque Compensation/1, [compensation_engine]  "engine torque compensation"

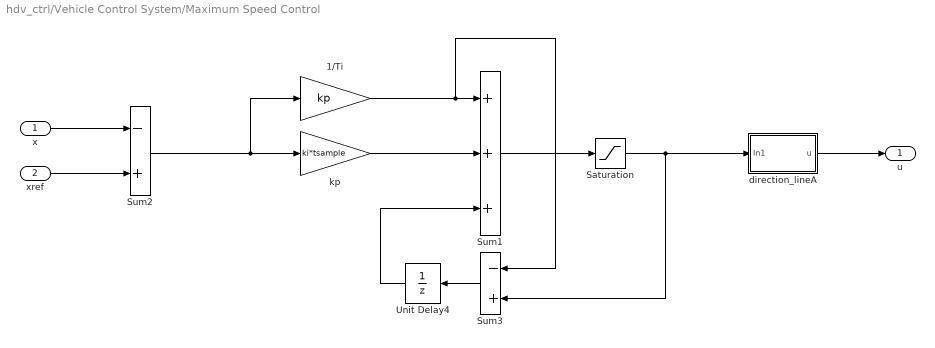
== system hdv_ctrl/Vehicle Control System/Maximum Speed Control ==
  x : Inport
  xref : Inport  Port=2
  1/Ti : Gain  Gain=kp  SaturateOnIntegerOverflow=on  OutDataTypeStr=Inherit: Same as input  ParamDataTypeStr=Inherit: Same as input
  Saturation : Saturate  UpperLimit=sat_pos  LowerLimit=sat_neg
  Sum1 : Sum  Inputs=+++  SaturateOnIntegerOverflow=on
  Sum2 : Sum  Inputs=-+  SaturateOnIntegerOverflow=on
  Sum3 : Sum  Inputs=-+  SaturateOnIntegerOverflow=on
  Unit Delay4 : UnitDelay  SampleTime=ts
  direction_lineA : Subsystem
  kp : Gain  Gain=ki*tsample  SaturateOnIntegerOverflow=on  OutDataTypeStr=Inherit: Same as input  ParamDataTypeStr=Inherit: Same as input
  u : Outport
  wires:
  xref/1 -> Sum2/2
  kp/1 -> Sum1/2
  1/Ti/1 -> Sum1/1, Sum3/1
  Sum3/1 -> Unit Delay4/1
  x/1 -> Sum2/1
  Sum1/1 -> Saturation/1
  Unit Delay4/1 -> Sum1/3
  Saturation/1 -> direction_lineA/1(In1), Sum3/2
  Sum2/1 -> kp/1, 1/Ti/1
  direction_lineA/1(u) -> u/1

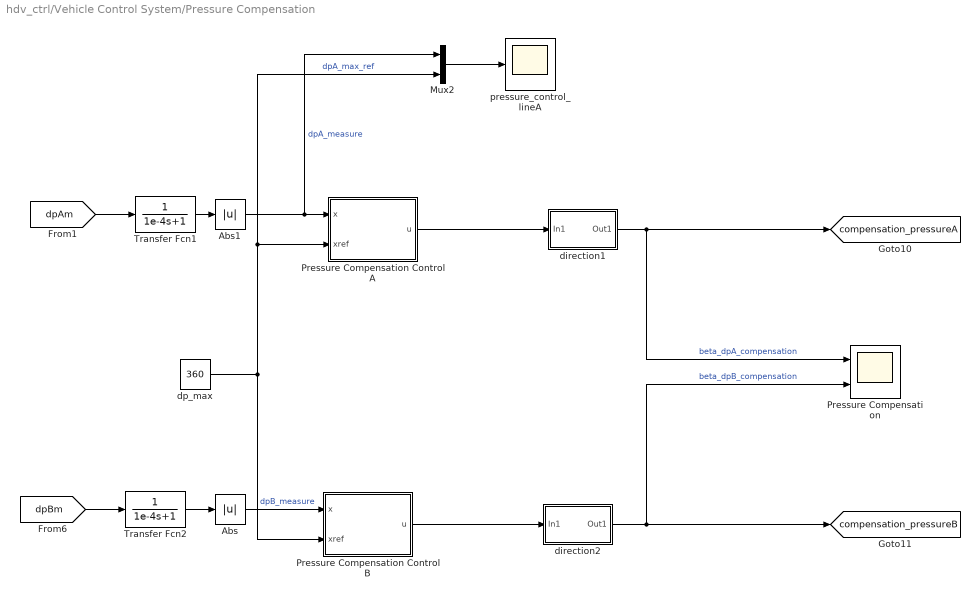
== system hdv_ctrl/Vehicle Control System/Pressure Compensation ==
  Abs : Abs  SaturateOnIntegerOverflow=off
  Abs1 : Abs  SaturateOnIntegerOverflow=off
  Mux2 : Mux  Inputs=2
  Pressure Compensation : Scope  NumInputPorts=2
      settings: SampleTime=tsample  ActiveDisplayYMinimum=-1  ActiveDisplayYMaximum=1
  Pressure Compensation Control A : Subsystem  mask{kp=0.00125, ki=0.02, ts=tsample, sat_pos=0, sat_neg=-1.64}
  Pressure Compensation Control B : Subsystem  mask{kp=0.00125, ki=0.02, ts=tsample, sat_pos=0, sat_neg=-1.64}
  Transfer Fcn1 : TransferFcn  Denominator=[1e-4 1]
  Transfer Fcn2 : TransferFcn  Denominator=[1e-4 1]
  direction1 : Subsystem
  direction2 : Subsystem
  dp_max : Constant  Value=360
  pressure_control_lineA : Scope
      settings: SampleTime=tsample  ActiveDisplayYMinimum=-53.40034  ActiveDisplayYMaximum=480.60302  DataLoggingVariableName=ScopeData6
  tag scope: compensation_pressureA=global, compensation_pressureB=global
  wires:
  Abs1/1 -> Mux2/1, Pressure Compensation Control A/1(x)  "dpA_measure"
  Transfer Fcn1/1 -> Abs1/1
  [dpBm] -> Transfer Fcn2/1
  dp_max/1 -> Pressure Compensation Control B/2(xref), Pressure Compensation Control A/2(xref), Mux2/2  "dpA_max_ref"
  direction1/1(Out1) -> [compensation_pressureA], Pressure Compensation/1  "beta_dpA_compensation"
  Mux2/1 -> pressure_control_lineA/1
  [dpAm] -> Transfer Fcn1/1
  Pressure Compensation Control B/1(u) -> direction2/1(In1)
  direction2/1(Out1) -> [compensation_pressureB], Pressure Compensation/2  "beta_dpB_compensation"
  Transfer Fcn2/1 -> Abs/1
  Pressure Compensation Control A/1(u) -> direction1/1(In1)
  Abs/1 -> Pressure Compensation Control B/1(x)  "dpB_measure"

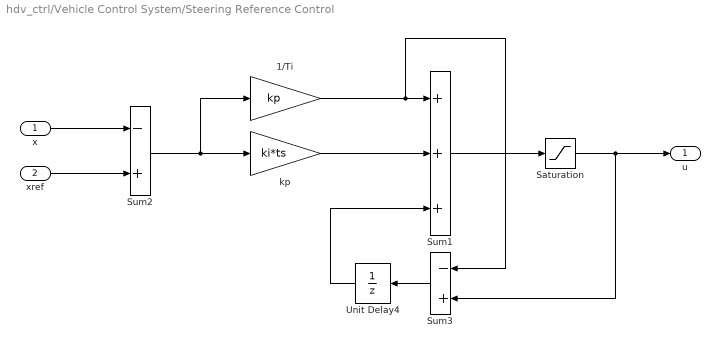
== system hdv_ctrl/Vehicle Control System/Steering Reference Control ==
  x : Inport
  xref : Inport  Port=2
  1/Ti : Gain  Gain=kp  SaturateOnIntegerOverflow=on  OutDataTypeStr=Inherit: Same as input  ParamDataTypeStr=Inherit: Same as input
  Saturation : Saturate  UpperLimit=sat_pos  LowerLimit=sat_neg
  Sum1 : Sum  Inputs=+++  SaturateOnIntegerOverflow=on
  Sum2 : Sum  Inputs=-+  SaturateOnIntegerOverflow=on
  Sum3 : Sum  Inputs=-+  SaturateOnIntegerOverflow=on
  Unit Delay4 : UnitDelay  SampleTime=tsample
  kp : Gain  Gain=ki*ts  SaturateOnIntegerOverflow=on  OutDataTypeStr=Inherit: Same as input  ParamDataTypeStr=Inherit: Same as input
  u : Outport
  wires:
  Saturation/1 -> Sum3/2, u/1
  Unit Delay4/1 -> Sum1/3
  Sum1/1 -> Saturation/1
  x/1 -> Sum2/1
  Sum3/1 -> Unit Delay4/1
  1/Ti/1 -> Sum3/1, Sum1/1
  Sum2/1 -> 1/Ti/1, kp/1
  kp/1 -> Sum1/2
  xref/1 -> Sum2/2

== system hdv_ctrl/Vehicle Control System/direction_lineLT ==
  In1 : Inport
  Abs1 : Abs  SaturateOnIntegerOverflow=off
  Product : Product
  Out1 : Outport
  wires:
  [direction_LT] -> Product/2
  In1/1 -> Abs1/1
  Product/1 -> Out1/1
  Abs1/1 -> Product/1

== system hdv_ctrl/Vehicle Control System/direction_lineRT ==
  In1 : Inport
  Abs : Abs  SaturateOnIntegerOverflow=off
  Product : Product
  Out1 : Outport
  wires:
  Product/1 -> Out1/1
  In1/1 -> Abs/1
  [direction_RT] -> Product/2
  Abs/1 -> Product/1

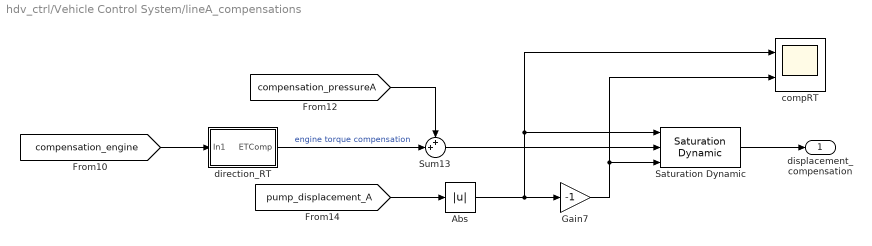
== system hdv_ctrl/Vehicle Control System/lineA_compensations ==
  Abs : Abs  SaturateOnIntegerOverflow=off
  Gain7 : Gain  Gain=-1
  Saturation Dynamic : sl_discontinuities/Saturation Dynamic  OutMin=[]  OutMax=[]  OutDataTypeStr=Inherit: Same as second input  OutDataType=fixdt(1, 16)  OutScaling=2^-10  DoSatur=off
  Sum13 : Sum  Inputs=++|
  compRT : Scope  NumInputPorts=2
      settings: SampleTime=tsample  ActiveDisplayYMinimum=-0.87768  ActiveDisplayYMaximum=2.34751  DataLoggingVariableName=ScopeData4
  direction_RT : Subsystem
  displacement_compensation : Outport
  wires:
  Saturation Dynamic/1 -> displacement_compensation/1
  Sum13/1 -> Saturation Dynamic/2
  Gain7/1 -> compRT/2, Saturation Dynamic/3
  [compensation_pressureA] -> Sum13/1
  [compensation_engine] -> direction_RT/1(In1)
  direction_RT/1(ETComp) -> Sum13/2  "engine torque compensation"
  [pump_displacement_A] -> Abs/1
  Abs/1 -> Saturation Dynamic/1, compRT/1, Gain7/1

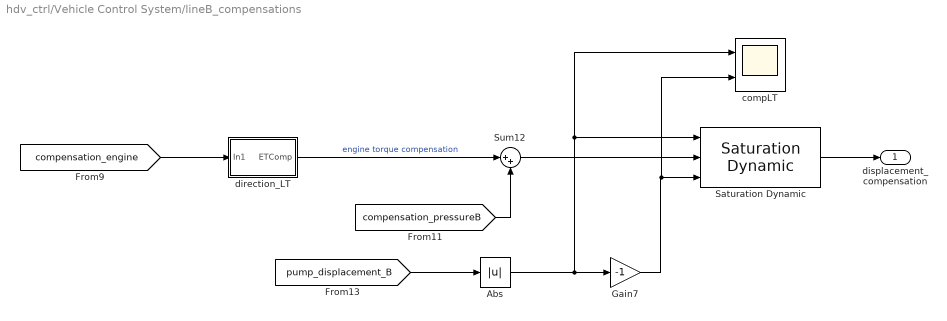
== system hdv_ctrl/Vehicle Control System/lineB_compensations  ==
  Abs : Abs  SaturateOnIntegerOverflow=off
  Gain7 : Gain  Gain=-1
  Saturation Dynamic : sl_discontinuities/Saturation Dynamic  OutMin=[]  OutMax=[]  OutDataTypeStr=Inherit: Same as second input  OutDataType=fixdt(1, 16)  OutScaling=2^-10  DoSatur=off
  Sum12 : Sum  Inputs=|++
  compLT : Scope  NumInputPorts=2
      settings: SampleTime=tsample  ActiveDisplayYMinimum=-1.80203  ActiveDisplayYMaximum=1.80203  DataLoggingVariableName=ScopeData5
  direction_LT : Subsystem
  displacement_compensation : Outport
  wires:
  [compensation_pressureB] -> Sum12/2
  Gain7/1 -> compLT/2, Saturation Dynamic/3
  [compensation_engine] -> direction_LT/1(In1)
  direction_LT/1(ETComp) -> Sum12/1  "engine torque compensation"
  [pump_displacement_B] -> Abs/1
  Sum12/1 -> Saturation Dynamic/2
  Saturation Dynamic/1 -> displacement_compensation/1
  Abs/1 -> Saturation Dynamic/1, compLT/1, Gain7/1

== system hdv_ctrl/external_load/loadA ==
  Rate Limiter : RateLimiter  RisingSlewLimit=tau_load_max/5  FallingSlewLimit=-tau_load_max/5  SampleTimeMode=inherited
  Saturation : Saturate  UpperLimit=abs(tau_load)  LowerLimit=-abs(tau_load)
  Step : Step  Time=5  FinalValue=tau_load  SampleTime=0
  Out1 : Outport
  wires:
  Saturation/1 -> Out1/1
  Rate Limiter/1 -> Saturation/1
  Step/1 -> Rate Limiter/1

== system hdv_ctrl/external_load/loadB ==
  Rate Limiter : RateLimiter  RisingSlewLimit=tau_load_max/5  FallingSlewLimit=-tau_load_max/5  SampleTimeMode=inherited
  Saturation : Saturate  UpperLimit=abs(tau_load)  LowerLimit=-abs(tau_load)
  Step : Step  Time=5  FinalValue=tau_load  SampleTime=0
  Out1 : Outport
  wires:
  Step/1 -> Rate Limiter/1
  Rate Limiter/1 -> Saturation/1
  Saturation/1 -> Out1/1

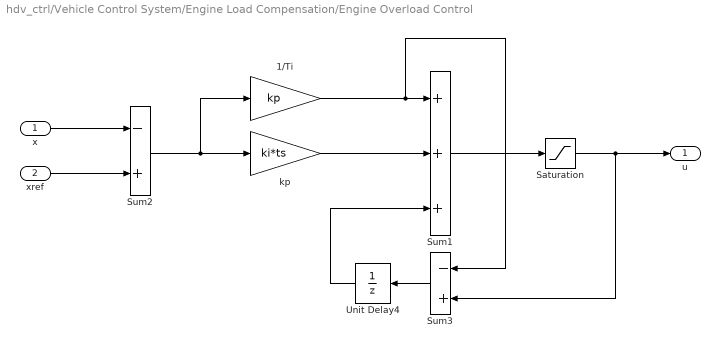
== system hdv_ctrl/Vehicle Control System/Engine Load Compensation/Engine Overload Control ==
  x : Inport
  xref : Inport  Port=2
  1/Ti : Gain  Gain=kp  SaturateOnIntegerOverflow=on  OutDataTypeStr=Inherit: Same as input  ParamDataTypeStr=Inherit: Same as input
  Saturation : Saturate  UpperLimit=sat_pos  LowerLimit=sat_neg
  Sum1 : Sum  Inputs=+++  SaturateOnIntegerOverflow=on
  Sum2 : Sum  Inputs=-+  SaturateOnIntegerOverflow=on
  Sum3 : Sum  Inputs=-+  SaturateOnIntegerOverflow=on
  Unit Delay4 : UnitDelay  SampleTime=tsample
  kp : Gain  Gain=ki*ts  SaturateOnIntegerOverflow=on  OutDataTypeStr=Inherit: Same as input  ParamDataTypeStr=Inherit: Same as input
  u : Outport
  wires:
  Saturation/1 -> Sum3/2, u/1
  Unit Delay4/1 -> Sum1/3
  Sum1/1 -> Saturation/1
  x/1 -> Sum2/1
  Sum3/1 -> Unit Delay4/1
  1/Ti/1 -> Sum3/1, Sum1/1
  Sum2/1 -> 1/Ti/1, kp/1
  kp/1 -> Sum1/2
  xref/1 -> Sum2/2

== system hdv_ctrl/Vehicle Control System/Maximum Speed Control/direction_lineA ==
  In1 : Inport
  Product : Product
  u : Outport
  wires:
  Product/1 -> u/1
  In1/1 -> Product/1
  [direction_SUM] -> Product/2

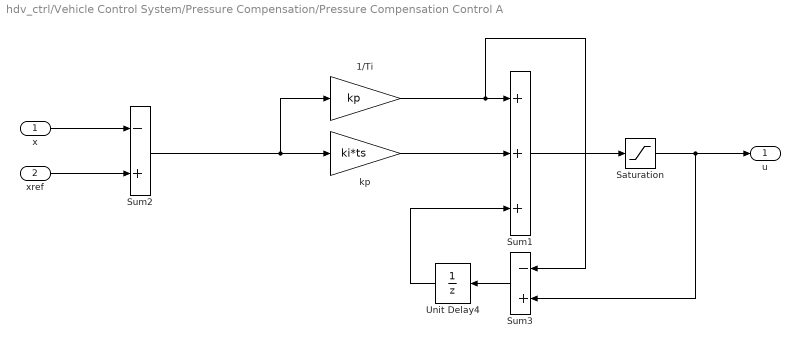
== system hdv_ctrl/Vehicle Control System/Pressure Compensation/Pressure Compensation Control A ==
  x : Inport
  xref : Inport  Port=2
  1/Ti : Gain  Gain=kp  SaturateOnIntegerOverflow=on  OutDataTypeStr=Inherit: Same as input  ParamDataTypeStr=Inherit: Same as input
  Saturation : Saturate  UpperLimit=sat_pos  LowerLimit=sat_neg
  Sum1 : Sum  Inputs=+++  SaturateOnIntegerOverflow=on
  Sum2 : Sum  Inputs=-+  SaturateOnIntegerOverflow=on
  Sum3 : Sum  Inputs=-+  SaturateOnIntegerOverflow=on
  Unit Delay4 : UnitDelay  SampleTime=tsample
  kp : Gain  Gain=ki*ts  SaturateOnIntegerOverflow=on  OutDataTypeStr=Inherit: Same as input  ParamDataTypeStr=Inherit: Same as input
  u : Outport
  wires:
  xref/1 -> Sum2/2
  kp/1 -> Sum1/2
  1/Ti/1 -> Sum1/1, Sum3/1
  Sum3/1 -> Unit Delay4/1
  x/1 -> Sum2/1
  Sum1/1 -> Saturation/1
  Unit Delay4/1 -> Sum1/3
  Saturation/1 -> u/1, Sum3/2
  Sum2/1 -> 1/Ti/1, kp/1

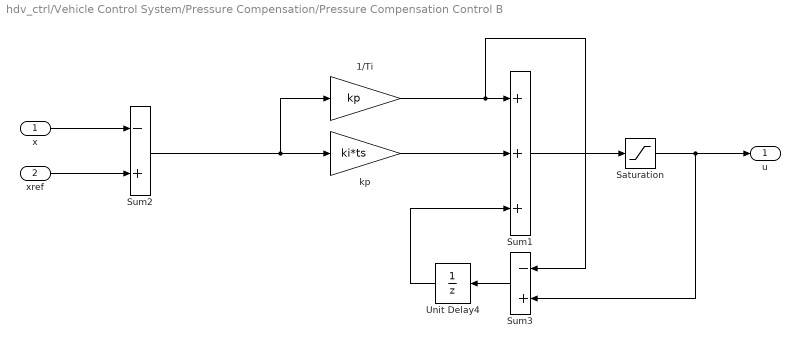
== system hdv_ctrl/Vehicle Control System/Pressure Compensation/Pressure Compensation Control B ==
  x : Inport
  xref : Inport  Port=2
  1/Ti : Gain  Gain=kp  SaturateOnIntegerOverflow=on  OutDataTypeStr=Inherit: Same as input  ParamDataTypeStr=Inherit: Same as input
  Saturation : Saturate  UpperLimit=sat_pos  LowerLimit=sat_neg
  Sum1 : Sum  Inputs=+++  SaturateOnIntegerOverflow=on
  Sum2 : Sum  Inputs=-+  SaturateOnIntegerOverflow=on
  Sum3 : Sum  Inputs=-+  SaturateOnIntegerOverflow=on
  Unit Delay4 : UnitDelay  SampleTime=tsample
  kp : Gain  Gain=ki*ts  SaturateOnIntegerOverflow=on  OutDataTypeStr=Inherit: Same as input  ParamDataTypeStr=Inherit: Same as input
  u : Outport
  wires:
  Saturation/1 -> Sum3/2, u/1
  Unit Delay4/1 -> Sum1/3
  Sum1/1 -> Saturation/1
  x/1 -> Sum2/1
  Sum3/1 -> Unit Delay4/1
  1/Ti/1 -> Sum3/1, Sum1/1
  Sum2/1 -> 1/Ti/1, kp/1
  kp/1 -> Sum1/2
  xref/1 -> Sum2/2

== system hdv_ctrl/Vehicle Control System/Pressure Compensation/direction1 ==
  In1 : Inport
  Product : Product
  Out1 : Outport
  wires:
  In1/1 -> Product/1
  Product/1 -> Out1/1
  [direction_RT] -> Product/2

== system hdv_ctrl/Vehicle Control System/Pressure Compensation/direction2 ==
  In1 : Inport
  Product : Product
  Out1 : Outport
  wires:
  Product/1 -> Out1/1
  In1/1 -> Product/1
  [direction_LT] -> Product/2

== system hdv_ctrl/Vehicle Control System/lineA_compensations/direction_RT ==
  In1 : Inport
  Product : Product
  ETComp : Outport
  wires:
  Product/1 -> ETComp/1
  In1/1 -> Product/1
  [direction_RT] -> Product/2

== system hdv_ctrl/Vehicle Control System/lineB_compensations /direction_LT ==
  In1 : Inport
  Product : Product
  ETComp : Outport
  wires:
  Product/1 -> ETComp/1
  In1/1 -> Product/1
  [direction_LT] -> Product/2

== matlab function hdv_ctrl/Vehicle Control System/Volumetric displacements calculation ==
  data: omega_e_rpm_ref input; Vd_p_R output; v_track1_ref input; v_track2_ref input; eta_vol_pump_right input; eta_vol_pump_left input; eta_vol_motor_right input; eta_vol_motor_left input; Vd_p_L output; v_track1_ref_cond output; v_track2_ref_cond output
function [Vd_p_R, Vd_p_L, v_track1_ref_cond, v_track2_ref_cond] = fcn(omega_e_rpm_ref, v_track1_ref, v_track2_ref, eta_vol_pump_right, eta_vol_pump_left, eta_vol_motor_right, eta_vol_motor_left)

n_tg = 41.4;
R_tg = 0.44056;
Vm_nom = 252.8;
Vp_nom = 147.2;
v_track_sum_max = 22;
v_track_diff_max = 11;

eta_vol_tot_right = eta_vol_pump_right*eta_vol_motor_right;
eta_vol_tot_left = eta_vol_pump_left*eta_vol_motor_left;

v_track_sum = v_track1_ref + v_track2_ref;
v_track_diff = v_track1_ref - v_track2_ref;

if v_track_sum >= v_track_sum_max
    v_track_sum = v_track_sum_max;
end

if v_track_sum <= -v_track_sum_max
    v_track_sum = -v_track_sum_max;
end

if v_track_diff >= v_track_diff_max
    v_track_diff = v_track_diff_max;
end

if v_track_diff <= -v_track_diff_max
    v_track_diff = -v_track_diff_max;
end

v_track1_ref_cond = 1/2*(v_track_sum + v_track_diff);
v_track2_ref_cond = 1/2*(v_track_sum - v_track_diff);

omega_l_1_ref_rpm = v_track1_ref_cond/3.6/R_tg/(2*pi)*60;
omega_l_2_ref_rpm = v_track2_ref_cond/3.6/R_tg/(2*pi)*60;

d1_ff_temp = abs(Vm_nom/Vp_nom/eta_vol_tot_right*omega_l_1_ref_rpm/omega_e_rpm_ref*n_tg);
d2_ff_temp = abs(Vm_nom/Vp_nom/eta_vol_tot_left*omega_l_2_ref_rpm/omega_e_rpm_ref*n_tg);

if d1_ff_temp >= 1
    Vd_p_R = 2 - 1/d1_ff_temp;
else
    Vd_p_R = d1_ff_temp;
end
if d2_ff_temp >= 1
    Vd_p_L = 2 - 1/d2_ff_temp;
else
    Vd_p_L = d2_ff_temp;
end
